simulink model "Test"  (R2015b)
settings: Solver=FixedStepDiscrete  SolverMode=SingleTasking  StartTime=0.0  StopTime=inf  RelTol=1e-3
libraries: simulink x2, arduinolib x2
settings Model: ExtModeTrigDuration=2  Creator=Druzhinin_Vasily  LastModifiedBy=Druzhinin_Vasily
settings OptimizationCC: DefaultParameterBehavior=Inlined  UseFloatMulNetSlope=on  InlineInvariantSignals=on  PassReuseOutputArgsAs=Individual arguments  ZeroExternalMemoryAtStartup=off  ZeroInternalMemoryAtStartup=off  NoFixptDivByZeroProtection=on  EfficientFloat2IntCast=on  OptimizeModelRefInitCode=on  LifeSpan=1  MaxStackSize=64
settings HardwareCC: ProdBitPerInt=16  ProdBitPerPointer=16  ProdLargestAtomicFloat=None  ProdWordSize=8  ProdHWDeviceType=Atmel->AVR
settings RTWCC: SystemTargetFile=ert.tlc  TemplateMakefile=ert_default_tmf  Description=Embedded Coder  GenerateReport=on  Toolchain=Arduino AVR v1.6.1  BuildConfiguration=Faster Runs  IncludeHyperlinkInReport=on  LaunchReport=on  GenerateTraceInfo=on  GenerateTraceReport=on  GenerateTraceReportSl=on  GenerateTraceReportSf=on  GenerateTraceReportEml=on  GenerateCodeMetricsReport=on
settings CodeAppCC: ForceParamTrailComments=on  IgnoreCustomStorageClasses=off  SimulinkDataObjDesc=on  CustomSymbolStrGlobalVar=rt$N$M  CustomSymbolStrType=$N$M  CustomSymbolStrFcn=$N$M$F  CustomSymbolStrMacro=$N$M  InsertBlockDesc=on
settings ERTTargetCC: IncludeMdlTerminateFcn=off  CombineSignalStateStructs=on  SupportNonFinite=off  SupportVariableSizeSignals=on  InlinedParameterPlacement=NonHierarchical  ERTFilePackagingFormat=CompactWithDataFile

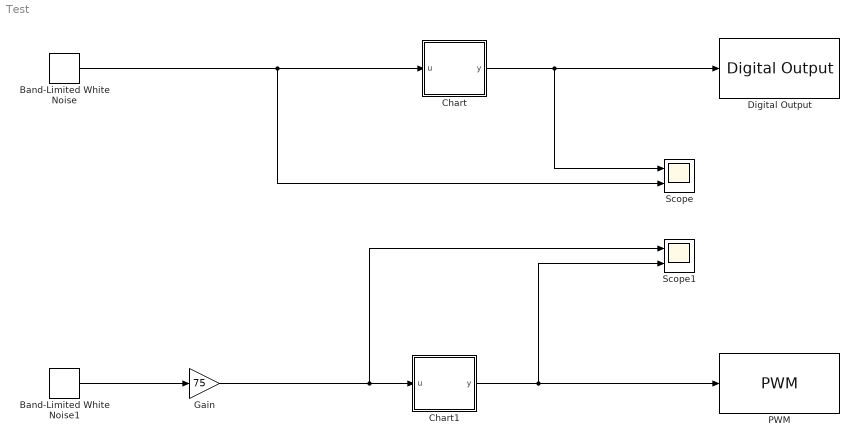
== system Test ==
  Band-Limited White Noise : simulink/Sources/Band-Limited White Noise  Cov=[1]  Ts=0.1  seed=[23341]
  Band-Limited White Noise1 : simulink/Sources/Band-Limited White Noise  Cov=[1]  Ts=0.5  seed=[123]
  Chart : Stateflow chart  TreatAsAtomicUnit=on
  Chart1 : Stateflow chart  TreatAsAtomicUnit=on
  Digital Output : arduinolib/Digital Output  pinNumber=9  blockPlatform=arduino
  Gain : Gain  Gain=75
  PWM : arduinolib/PWM  pinNumber=5  blockPlatform=arduino
  Scope : Scope  NumInputPorts=2
  Scope1 : Scope  NumInputPorts=2
  wires:
  Chart/1(y) -> Scope/1, Digital Output/1
  Band-Limited White Noise/1 -> Scope/2, Chart/1(u)
  Band-Limited White Noise1/1 -> Gain/1
  Chart1/1(y) -> Scope1/2, PWM/1
  Gain/1 -> Chart1/1(u), Scope1/1

== stateflow chart Test/Chart1 ==
  state Off
    entry: y= u*(-1)
  state On
    entry: y = u*1
  (default) -> On
  On -> Off [order 1] : [u<0]
  Off -> On [order 1] : [u>0]
  Off -> Off [order 2] : [y~=u]
  On -> On [order 2] : [u~=y]
  data: u input; y output

== stateflow chart Test/Chart ==
  state Off
    entry: y=0
  state On
    entry: y = 1
  (default) -> On
  On -> Off : [u<0]
  Off -> On : [u>0]
  data: u input; y output
